simulink model "Microgrid_PV_WG_Bat_EV_j"  (R2023b)
settings: Solver=VariableStepAuto  StartTime=0.0  StopTime=1  RelTol=1e-3
undefined symbols (not defined in the file or in its folder): Acid, Ion, Lead, Lithium
libraries: slpidlib x35, spsabctodq0Lib x23, spsSeriesRLCBranchLib x19, spsCurrentMeasurementLib x13, spsVoltageMeasurementLib x11, spsThreePhaseVIMeasurementLib x10, spsPLL3phLib x9, spsThreePhaseSeriesRLCBranchLib x9, spsPower3phInstantaneousLib x8, spsIGBTDiodeLib x8, spsUniversalBridgeLib x7, spsPWMGeneratorDCDCLib x6
(part 1 of 5)
settings Model: SimulationMode=accelerator  Creator=USER  LastModifiedBy=User

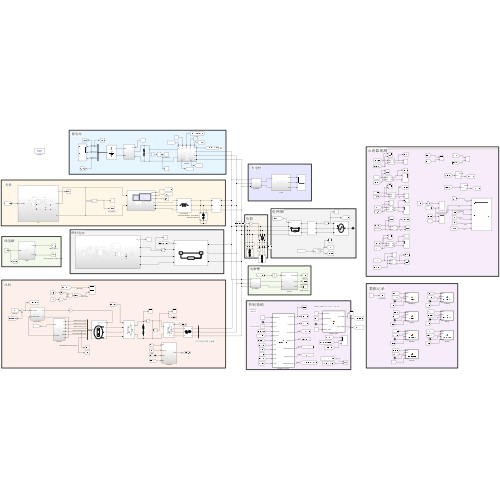
[thumbnail: Simulink's stored preview of the top-level diagram]
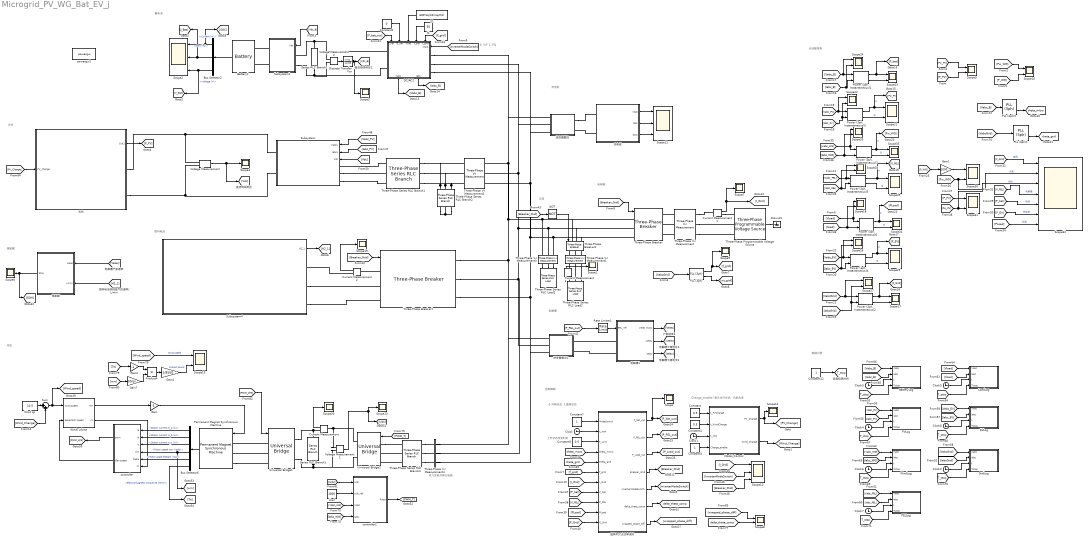
== system Microgrid_PV_WG_Bat_EV_j ==
  note: Change_enable:1表示允许光伏、风机改变
  note: :0 并网状态
      | :1 离网状态
  note: 蓄电池
  note: 储氢罐
  note: 充电桩
  note: 电解槽
  note: 燃料电池
  note: 0: V/F
      | 1: PQ
  note: 光伏
  note: 风力发电并网主电路
  note: 风机
  note: 示波器观测
  note: 数据记录
  note: 工作状态改变时刻
  note: 控制策略
  note: 负荷
  note: 电网侧
  Battery1 : spsBatteryLib/Battery  BatType=Lithium-Ion  ShowTempParam=off  ThermalPreset=no  ShowAgeParam=off  NomV=600  NomQ=10000  SOC=50  Batt_Tr=30  PresetModel=on  MaxQ=10000  MinV=450  FullV=698.3923  Dis_rate=4347.8261  R=0.0006  Normal_OP=9043.4783  expZone="[648.2315      491.3043]"  current=[6.5 13 32.5]  Units=Time  Tci=20  NomT=20  T2=-30  MaxQ2=4.8  FullV2=7.1  Normal_OP2=5.655  expZone2="[6.58           1]"  Rca=0.6  ti=2000  Dp=0  Neq0=0  Tsim=1e6  Ta1=25  Qeol=5.4*0.9  Reol=0.013333*1.2  Char_age=[2.3478, 3]  Dis_age=[2.3478, 10]  N1=1500  N2=10500  N3=1000  N4=1400  Ta2=45  N5=950
  BatteryLog : MATLAB Function  TreatAsAtomicUnit=on  SystemSampleTime=1e-5
  Bus Selector2 : BusSelector  OutputSignals=SOC (%),Current (A),Voltage (V)
  Bus Selector6 : BusSelector  OutputSignals=Stator current is_a (A),Stator current is_b (A),Stator current is_c (A),Rotor speed wm (rad/s),Rotor angle thetam (rad),Electromagnetic torque Te (N*m)
  Clock{,1..8} (9 alike) : Clock
  Constant : Constant  Value=0.5
  Constant1 : Constant  Value=0.5
  Constant12 : Constant
  Constant2 : Constant  Value=0
  Constant3 : Constant
  Constant5 : Constant  Value=0.5
  Constant7 : Constant
  Current Measurement{,1..3} (4 alike) : spsCurrentMeasurementLib/Current Measurement  PhasorSimulation=off  OutputType=Complex  PSBequivalent=0
  DC/AC2 : Subsystem
      settings: PortSchema="{\"entries\":[{\"content\":{\"sides\":[{\"content\":{\"connectorIds\":[\"LConn1\",\"LConn2\"]},\"type\":\"ConnectorPlacement.EquallySpacedRectSide\",\"uuid\":\"3c25f3ef-dfc4-4171-a66c-34d02ac02d8c\"},{\"content\":{\"connectorIds\":[\"In6\",\"RConn1\",\"RConn2\",\"RConn3\"],\"side\":\"RIGHT\"},\"type\":\"ConnectorPlacement.EquallySpacedRectSide\",\"uuid\":\"e6dce20c-09a8-4093-a340-4a6433e2abb5\"},{\"content\":{\"connectorIds\":[\"In1\",\"In2\",\"In3\",\"In4\",\"In5\"],\"side\":\"TOP\"},\"type\":\"ConnectorPlacement.EquallySpacedRectSide\",\"uuid\":\"9a728458-db9e-49f2-aa6e-65bbdb48c66f\"},{\"content\":{\"connectorIds\":[\"Out1\",\"Out2\"],\"side\":\"BOTTOM\"},\"type\":\"ConnectorPlacement.EquallySpacedRectSide\",\"uuid\":\"1b603170-02ae-4700-b32b-0d723ac1cdee\"}]},\"type\":\"ConnectorPlacement.EquallySpacedConnector\",\"uuid\":\"ee4962e9-610e-4348-91fe-b672627aeb34\"}],\"packageUris\":[\"http://schema.mathworks.com/mf0/Connector/R2020b\"],\"version\":\"1.0\"}"
  Discrete Transfer Fcn : DiscreteTransferFcn  Numerator=[0.02]  Denominator=[1 -0.98]
  EVLog : MATLAB Function  TreatAsAtomicUnit=on  SystemSampleTime=1e-5
  Gain : Gain  Gain=-1
  Gain1 : Gain  Gain=1000
  Gain2 : Gain  Gain=-1
  Gain4 : Gain  Gain=1/9550
  Gain7 : Gain  Gain=30/pi
  GridLog : MATLAB Function  TreatAsAtomicUnit=on  SystemSampleTime=1e-5
  Ground1 : spsGroundLib/Ground  LConnTagsString=a
  LoadLog : MATLAB Function  TreatAsAtomicUnit=on  SystemSampleTime=1e-5
  Model_Control : MATLAB Function  TreatAsAtomicUnit=on
  NOT : Logic  Operator=NOT  IconShape=distinctive  AllPortsSameDT=off  OutDataTypeStr=boolean
  PELLog : MATLAB Function  TreatAsAtomicUnit=on  SystemSampleTime=1e-5
  PLL (3ph) : spsPLL3phLib/PLL (3ph)  Fmin=0.0001  Par_Init=[0, 50]  ParK=[180, 3200, 1]  TcD=1e-6  MaxRateChangeFreq=100  FilterCutOffFreq=25  Ts=0  AGC=on
  PLL (3ph)1 : spsPLL3phLib/PLL (3ph)  Fmin=45  Par_Init=[0, 50]  ParK=[180, 3200, 1]  TcD=1e-4  MaxRateChangeFreq=12  FilterCutOffFreq=25  Ts=0  AGC=on
  PLL (3ph)2 : spsPLL3phLib/PLL (3ph)  Fmin=45  Par_Init=[0, 50]  ParK=[180, 3200, 1]  TcD=1e-4  MaxRateChangeFreq=12  FilterCutOffFreq=25  Ts=0  AGC=on
  PVLog : MATLAB Function  TreatAsAtomicUnit=on  SystemSampleTime=1e-5
  Permanent Magnet Synchronous Machine : spsPermanentMagnetSynchronousMachineLib/Permanent Magnet Synchronous Machine  NbPhases=3  FluxDistribution=Sinusoidal  RotorType=Round  MechanicalLoad=Torque Tm  PresetModel=No  ShowDetailedParameters=on  MeasurementBus=off  Resistance=0.025  Inductance=8.5e-3  dqInductances=[8.5e-3,8.5e-3]  La=0.0036  MachineConstant=Flux linkage established by magnets (V.s)  Flux=3.88889  VoltageCst=8464.3995  TorqueCst=70  Flat=120  Mechanical=[60 0.078 12]  PolePairs=4  InitialConditions=[0,0, 0,0]  InitialConditions5ph=[0 0 0 0 0 0]  RefAngle=90 degrees behind phase A axis (modified Park)  IterativeDiscreteModel=Trapezoidal non iterative  TsBlock=-1  TsPowergui=0
  Power (3ph, Instantaneous){1..7} (7 alike) : spsPower3phInstantaneousLib/Power (3ph, Instantaneous)
  Product4 : Product
  Rate Limiter1 : RateLimiter  RisingSlewLimit=100e5  FallingSlewLimit=-100e5
  Scope{,1,3..7,12..13,15,20} (11 alike) : Scope
  Scope10 : Scope  NumInputPorts=3
  Scope11 : Scope  NumInputPorts=3
  Scope{8..9,16..19,21..31,33..35} (20 alike) : Scope  NumInputPorts=2
  Scope2 : Scope  NumInputPorts=3
  Scope32 : Scope  NumInputPorts=7
  Series RLC Branch1 : spsSeriesRLCBranchLib/Series RLC Branch  LConnTagsString=__new0  RConnTagsString=__new0  BranchType=RC  Resistance=0.05  Inductance=1e-3  SetiL0=off  InitialCurrent=0  Capacitance=1e-2  Setx0=on  InitialVoltage=1800  Measurements=None
  Series RLC Branch2 : spsSeriesRLCBranchLib/Series RLC Branch  LConnTagsString=__new0  RConnTagsString=__new0  BranchType=RC  Resistance=0.05  Inductance=1e-3  SetiL0=off  InitialCurrent=0  Capacitance=7e-2  Setx0=on  InitialVoltage=1000  Measurements=None
  Subsystem : Subsystem
  Subsystem1 : Subsystem
  Subsystem4 : Subsystem
  Sum : Sum  Inputs=|++
  Three-Phase Programmable Voltage Source : spsThreePhaseProgrammableVoltageSourceLib/Three-Phase Programmable Voltage Source  PositiveSequence="[600  0 50]"  VariationEntity=None  VariationType=Table of time-amplitude pairs  VariationTypeAlt=Ramp  VariationStep=-5  VariationRate=100  VariationMagnitude=0.3  VariationFrequency=2  VariationTiming=[0.5 1]  VariationPhaseA=off  Amplitudes=[1 0.8 1.2 1.0]  TimeValues=[0 0.1 0.15 0.2]  HarmonicGeneration=off  HarmonicA=[3 0.2 -25 0]  HarmonicB=[2 0.15 35 2]  Timing="[0.05  3]"  BusType=swing  Pref=0  Qref=0  Qmin=-inf  Qmax=inf
  Three-Phase Series RLC Branch1 : spsThreePhaseSeriesRLCBranchLib/Three-Phase Series RLC Branch  LConnTagsString=A|B|C  RConnTagsString=A|B|C  BranchType=L  Resistance=0.1  Inductance=3e-3  Capacitance=1e-6  Measurements=None
  Three-Phase Series RLC Branch2 : spsThreePhaseSeriesRLCBranchLib/Three-Phase Series RLC Branch  LConnTagsString=A|B|C  RConnTagsString=A|B|C  BranchType=RC  Resistance=0.01  Inductance=1e-5  Capacitance=1e-5  Measurements=None
  Three-Phase Series RLC Branch3 : spsThreePhaseSeriesRLCBranchLib/Three-Phase Series RLC Branch  LConnTagsString=A|B|C  RConnTagsString=A|B|C  BranchType=RL  Resistance=0.05  Inductance=7e-3  Capacitance=1e-6  Measurements=None
  Three-Phase Series RLC Load1 : spsThreePhaseSeriesRLCLoadLib/Three-Phase Series RLC Load  LConnTagsString=A|B|C  Configuration=Y (grounded)  NominalVoltage=380  Vabc=[600 600 600]  Vabcp=[1e3 1e3 1e3]  NominalFrequency=50  UnbalancedPower=on  ActivePower=150e3  InductivePower=0  CapacitivePower=0  Pabc=[33e4 33e4 33e4]  QLabc=[100 90 110]  QCabc=[100 90 110]  Pabcp=[10e3 9e3 11e3]  QLabcp=[100 90 110]  QCabcp=[100 90 110]  Measurements=None  LoadType=constant PQ
  Three-Phase Series RLC Load2 : spsThreePhaseSeriesRLCLoadLib/Three-Phase Series RLC Load  LConnTagsString=A|B|C  Configuration=Y (grounded)  NominalVoltage=380  Vabc=[600 600 600]  Vabcp=[1e3 1e3 1e3]  NominalFrequency=50  UnbalancedPower=on  ActivePower=150e3  InductivePower=0  CapacitivePower=0  Pabc=[41e4 41e4 41e4]  QLabc=[100 90 110]  QCabc=[100 90 110]  Pabcp=[10e3 9e3 11e3]  QLabcp=[100 90 110]  QCabcp=[100 90 110]  Measurements=None  LoadType=constant PQ
  Three-Phase V-I Measurement : spsThreePhaseVIMeasurementLib/Three-Phase V-I Measurement  VoltageMeasurement=phase-to-ground  SetLabelV=on  LabelV=VabcGrid  Vpu=off  VpuLL=off  CurrentMeasurement=yes  SetLabelI=on  LabelI=IabcGrid  Ipu=off  Pbase=100e6  Vbase=500e3  OutputType=Complex  PhasorSimulation=off  PSBequivalent=0
  Three-Phase V-I Measurement1 : spsThreePhaseVIMeasurementLib/Three-Phase V-I Measurement  VoltageMeasurement=phase-to-ground  SetLabelV=on  LabelV=Vload1  Vpu=off  VpuLL=off  CurrentMeasurement=yes  SetLabelI=on  LabelI=Iload1  Ipu=off  Pbase=100e6  Vbase=500e3  OutputType=Complex  PhasorSimulation=off  PSBequivalent=0
  Three-Phase V-I Measurement2 : spsThreePhaseVIMeasurementLib/Three-Phase V-I Measurement  VoltageMeasurement=phase-to-ground  SetLabelV=on  LabelV=Vabc_PV  Vpu=off  VpuLL=off  CurrentMeasurement=yes  SetLabelI=on  LabelI=Iabc_PV  Ipu=off  Pbase=100e6  Vbase=500e3  OutputType=Complex  PhasorSimulation=off  PSBequivalent=0
  Three-Phase V-I Measurement3 : spsThreePhaseVIMeasurementLib/Three-Phase V-I Measurement  VoltageMeasurement=phase-to-ground  SetLabelV=on  LabelV=Vload  Vpu=off  VpuLL=off  CurrentMeasurement=yes  SetLabelI=on  LabelI=Iload  Ipu=off  Pbase=100e6  Vbase=500e3  OutputType=Complex  PhasorSimulation=off  PSBequivalent=0
  Three-Phase V-I Measurement4 : spsThreePhaseVIMeasurementLib/Three-Phase V-I Measurement  VoltageMeasurement=phase-to-ground  SetLabelV=on  LabelV=Vabc_WG  Vpu=off  VpuLL=off  CurrentMeasurement=yes  SetLabelI=on  LabelI=Iabc_WG  Ipu=off  Pbase=100e6  Vbase=500e3  OutputType=Complex  PhasorSimulation=off  PSBequivalent=0
  Three-Phase Breaker : spsThreePhaseBreakerLib/Three-Phase Breaker  InitialState=closed  SwitchA=on  SwitchB=on  SwitchC=on  SwitchTimes=0.2  External=on  BreakerResistance=0.0001  SnubberResistance=1e9  SnubberCapacitance=inf  Measurements=Breaker voltages and currents
  Three-Phase Breaker1 : spsThreePhaseBreakerLib/Three-Phase Breaker  InitialState=closed  SwitchA=on  SwitchB=on  SwitchC=on  SwitchTimes=0.5  External=on  BreakerResistance=0.01  SnubberResistance=1e6  SnubberCapacitance=inf  Measurements=None
  Three-Phase Breaker2 : spsThreePhaseBreakerLib/Three-Phase Breaker  InitialState=closed  SwitchA=on  SwitchB=on  SwitchC=on  SwitchTimes=0.2  External=on  BreakerResistance=0.0001  SnubberResistance=1e9  SnubberCapacitance=inf  Measurements=Breaker voltages and currents
  Universal Bridge1 : spsUniversalBridgeLib/Universal Bridge  Arms=3  SnubberResistance=1e5  SnubberCapacitance=inf  Device=IGBT / Diodes  Ron=1e-3  Lon=0  ForwardVoltages="[  0  0  ]"  ForwardVoltage=0  GTOparameters=[ 10e-6 , 20e-6 ]  IGBTparameters=[ 1e-6 , 2e-6 ]  Measurements=None  Measurements_2=None  converterType=Rectifier
  Universal Bridge2 : spsUniversalBridgeLib/Universal Bridge  Arms=3  SnubberResistance=1e5  SnubberCapacitance=inf  Device=IGBT / Diodes  Ron=1e-3  Lon=0  ForwardVoltages="[  0  0  ]"  ForwardVoltage=0  GTOparameters=[ 10e-6 , 20e-6 ]  IGBTparameters=[ 1e-6 , 2e-6 ]  Measurements=None  Measurements_2=None  converterType=Rectifier
  Uref : Constant  Value=1800
  V1 : Constant  Value=600*sqrt(2)/sqrt(3)
  Voltage Measurement : spsVoltageMeasurementLib/Voltage Measurement  PhasorSimulation=off  OutputType=Complex  PSBequivalent=0
  Voltage Measurement1 : spsVoltageMeasurementLib/Voltage Measurement  PhasorSimulation=off  OutputType=Complex  PSBequivalent=0
  Voltage Measurement2 : spsVoltageMeasurementLib/Voltage Measurement  PhasorSimulation=off  OutputType=Complex  PSBequivalent=0
  Wind sp : Constant  Value=10.5
  WindLog : MATLAB Function  TreatAsAtomicUnit=on  SystemSampleTime=1e-5
  WindTurbine : Subsystem
  controller : Subsystem
  controller2 : Subsystem
  f1 : Constant  Value=50
  powergui1 : sps_lib/powergui  Priority=1  SimulationMode=Discrete  SampleTime=1e-6  frequency=60  Iterations=50  frequencyindice=0  Pbase=100e6  ErrMax=1e-4  UnitsV=kV  UnitsW=MW  buscounter=0  FunctionMessages=off  echomessages=off  EnableUseOfTLC=off  CurrentSourceSwitches=off  DisableSnubberDevices=off  DisableRonSwitches=off  DisableVfSwitches=off  DisplayEquations=off  AutomaticDiscreteSolvers=off  SolverType=Tustin/Backward Euler (TBE)  Interpol=off  ExternalGateDelay=off  methode=off  Ts=100  x0status=blocks  SPID=on  SwTol=0  HookPort=off  NonlinearTolerance=1e-4  nMaxIteration=100  ContinueOnMaxIteration=off  RestoreLinks=warning  ResistiveCurrentMeasurement=off  Frange=[0:2:500]  Ylog=off  Xlog=on  ShowGrid=off  save=off  variable=ZData  structure=0  ZoomFFT=off  StartTime=0.0  cycles=1  DisplayStyle=1  fundamental=60  FreqAxis=off  MaxFrequency=1000  frequencyindicesteady=1  RmsSteady=1  display=off
  储氢罐 : Subsystem
  充电桩 : Subsystem
      settings: PortSchema="{\"entries\":[{\"content\":{\"sides\":[{\"content\":{\"connectorIds\":[\"Out1\",\"Out2\",\"Out3\"]},\"type\":\"ConnectorPlacement.EquallySpacedRectSide\",\"uuid\":\"de89acf6-4bf1-40b6-9ccd-ec8106de39fd\"},{\"content\":{\"connectorIds\":[\"RConn1\",\"RConn2\"],\"side\":\"RIGHT\"},\"type\":\"ConnectorPlacement.EquallySpacedRectSide\",\"uuid\":\"d03cc6c4-9473-47ce-91a0-26eb3774d9eb\"},{\"content\":{\"side\":\"TOP\"},\"type\":\"ConnectorPlacement.EquallySpacedRectSide\",\"uuid\":\"dff31fb8-dbf6-4b34-953b-d6d002de7265\"}]},\"type\":\"ConnectorPlacement.EquallySpacedConnector\",\"uuid\":\"fa66b497-f06b-485d-a451-c3139dd511e8\"}],\"packageUris\":[\"http://schema.mathworks.com/mf0/Connector/R2020b\"],\"version\":\"1.0\"}"
  光伏 : Subsystem
  电解槽1 : Subsystem
  脱网PCC点功率调节 : MATLAB Function  TreatAsAtomicUnit=on  SystemSampleTime=1e-5
  逆变器整流 : Subsystem
      settings: RTWSystemCode=Inline
  逆变器整流1 : Subsystem
      settings: RTWSystemCode=Inline
  tag scope: T_stop=global, delta_theta_comp=global, theta_grid=global, theta_micro=global
  wires:
  Discrete Transfer Fcn/1 -> Scope3/1, [Vdc_B]
  Bus Selector2/2 -> Scope2/2, [I_Bat]  "<Current (A)>"
  [Vdc_B] -> Subsystem1/1(Vdc)
  Bus Selector2/1 -> Scope2/1, [SOC]  "<SOC (%)>"
  Voltage Measurement2/1 -> Discrete Transfer Fcn/1
  Bus Selector2/3 -> Scope2/3, [V_Bat]  "<Voltage (V)>"
  Battery1/1 -> Bus Selector2/1
  [Velec] -> 储氢罐/1(Velec)
  [H2_1] -> 储氢罐/2(L/min)
  储氢罐/1(SOH) -> Scope6/1, [SOH]
  充电桩/2(Ibat) -> Scope11/2
  充电桩/3(SOC) -> Scope11/3
  充电桩/1(Vbat) -> Scope11/1
  电解槽1/3(Ielec) -> [Ielec]
  电解槽1/1(Velec mol/s) -> [Velec]
  电解槽1/2(Uelec) -> [Uelec]
  [P_PEL_out] -> Rate Limiter1/1
  Rate Limiter1/1 -> 电解槽1/1(PEL_ref)
  Subsystem4/1(H2_1) -> [H2_1]
  [VabcGrid] -> PLL (3ph)/1
  PLL (3ph)/1 -> Scope5/1, [f_grid]
  PLL (3ph)/2 -> [wt_grid]
  Current Measurement1/1 -> Scope7/1, [I_Grid]
  [Breaker_Grid] -> Three-Phase Breaker/1
  DC/AC2/1(Vabc) -> [Vabc_B]
  f1/1 -> DC/AC2/4(f_set)
  [P_bat_out] -> DC/AC2/1(P_ref)
  [InverterModeSwitch] -> DC/AC2/6(Input)
  V1/1 -> DC/AC2/3(Vset)
  [f_grid] -> DC/AC2/5(f_grid)
  Constant2/1 -> DC/AC2/2(Q_ref)
  DC/AC2/2(Iabc) -> [Iabc_B]
  [Breaker_Grid] -> Three-Phase Breaker1/1
  Constant/1 -> Model_Control/1(t_PVChange)
  Model_Control/1(PV_Change) -> [PV_Change], Scope12/1
  Model_Control/2(Wind_Change) -> [Wind_Change]
  Current Measurement2/1 -> Scope15/1
  "Power (3ph, Instantaneous)3"/1 -> [Pw_PV], Scope21/1  "P"
  [Iabc_PV] -> Scope22/2, "Power (3ph, Instantaneous)3"/2
  "Power (3ph, Instantaneous)3"/2 -> Scope21/2  "Q"
  [Vabc_PV] -> Scope22/1, "Power (3ph, Instantaneous)3"/1
  [Iabc_B] -> Scope24/2, "Power (3ph, Instantaneous)1"/2
  [Vabc_B] -> Scope24/1, "Power (3ph, Instantaneous)1"/1
  "Power (3ph, Instantaneous)1"/2 -> Scope23/2
  "Power (3ph, Instantaneous)1"/1 -> [P_bat], Scope23/1
  [Vabc_EV] -> Scope26/1, "Power (3ph, Instantaneous)4"/1
  "Power (3ph, Instantaneous)4"/2 -> Scope25/2  "Q"
  "Power (3ph, Instantaneous)4"/1 -> [P_EV], Scope25/1  "P"
  [Iabc_EV] -> Scope26/2, "Power (3ph, Instantaneous)4"/2
  [IabcGrid] -> Scope27/2, "Power (3ph, Instantaneous)2"/2
  "Power (3ph, Instantaneous)2"/1 -> [P_Grid], Scope17/1
  [VabcGrid] -> Scope27/1, "Power (3ph, Instantaneous)2"/1
  "Power (3ph, Instantaneous)2"/2 -> Scope17/2
  "Power (3ph, Instantaneous)5"/2 -> Scope29/2  "Q"
  [Vabc_PEL] -> Scope28/1, "Power (3ph, Instantaneous)5"/1
  [Iabc_PEL] -> Scope28/2, "Power (3ph, Instantaneous)5"/2
  "Power (3ph, Instantaneous)5"/1 -> [P_PEL], Scope29/1  "P"
  [P_Grid] -> Scope32/1  "电网"
  [Pw_WG] -> Scope32/2, Scope30/2  "风机"
  [P_PEL] -> Scope32/4  "电解槽"
  [P_EV] -> Scope32/6  "充电桩"
  Gain1/1 -> Scope30/1
  [Pw_PV] -> Scope32/3, Scope31/2  "光伏"
  [P_bat] -> Scope32/5  "电池"
  [P_PV] -> Scope31/1
  [P_WG] -> Gain1/1
  "Power (3ph, Instantaneous)7"/1 -> Scope35/1, [Pw_WG]  "P"
  [Iabc_WG] -> Scope33/2, "Power (3ph, Instantaneous)7"/2
  [Vabc_WG] -> Scope33/1, "Power (3ph, Instantaneous)7"/1
  "Power (3ph, Instantaneous)7"/2 -> Scope35/2  "Q"
  [Pw_PV] -> Scope9/1
  [P_PV] -> Scope9/2
  [Pw_WG] -> Scope16/1
  [P_WG] -> Scope16/2
  "Power (3ph, Instantaneous)6"/1 -> Scope34/1, [PLoad]  "P"
  [Vload] -> Scope18/1, "Power (3ph, Instantaneous)6"/1
  [Iload] -> Scope18/2, "Power (3ph, Instantaneous)6"/2
  "Power (3ph, Instantaneous)6"/2 -> Scope34/2  "Q"
  [PLoad] -> Scope32/7  "负载"
  [PLoad] -> 脱网PCC点功率调节/10(PLoad)
  [P_Grid] -> 脱网PCC点功率调节/11(P_Grid)
  [P_bat] -> 脱网PCC点功率调节/8(P_bat)
  [P_PEL] -> 脱网PCC点功率调节/9(P_PEL)
  [I_Grid] -> Scope10/1
  [InverterModeSwitch] -> Scope10/2
  [Breaker_Grid] -> Scope10/3
  脱网PCC点功率调节/3(P_Load_out) -> [P_Load_out]
  [Iabc_PV] -> Subsystem/2(IabcL)
  [Vabc_PV] -> Subsystem/1(VabcL)
  光伏/1(Out1) -> [P_PV]
  Voltage Measurement/1 -> Scope4/1, [Vdc]
  [Vdc] -> Subsystem/3(Vdc)
  controller/2(Gen speed) -> WindTurbine/2(Generator speed)
  [Wind_Change] -> Sum/2
  Current Measurement/1 -> Scope20/1
  Bus Selector6/6 -> [Te]  "<Electromagnetic torque Te (N*m)>"
  [Iabc_WG] -> controller2/4(Iabc)
  Voltage Measurement1/1 -> [Udc], Scope13/1
  Gain/1 -> Permanent Magnet Synchronous Machine/1
  [Udc] -> controller2/1(Udc)
  Bus Selector6/3 -> controller/3(ic)  "<Stator current is_c (A)>"
  Gain4/1 -> Scope19/2  "Output power"
  WindTurbine/1(Tm) -> Gain/1
  [Vabc_WG] -> controller2/3(Vabc)
  Bus Selector6/4 -> [wm], controller/4(wm)  "<Rotor speed wm (rad/s)>"
  Permanent Magnet Synchronous Machine/1 -> Bus Selector6/1
  Gain7/1 -> Product4/2
  [PWM_T] -> Universal Bridge2/1
  Sum/1 -> WindTurbine/1(Wind speed), [Wind_speed]
  controller/1(pwm) -> [PWM_WG]
  [PWM_WG] -> Universal Bridge1/1
  [wm] -> Gain7/1
  [Wind_speed] -> Scope19/1  "Wind speed"
  Bus Selector6/1 -> controller/1(ia)  "<Stator current is_a (A)>"
  Gain2/1 -> Product4/1
  Bus Selector6/5 -> controller/5(theta)  "<Rotor angle thetam (rad)>"
  Bus Selector6/2 -> controller/2(ib)  "<Stator current is_b (A)>"
  WindTurbine/2(n*) -> controller/6(n*)
  Wind sp/1 -> Sum/1
  Product4/1 -> Gain4/1
  controller2/1(Pulse) -> [PWM_T]
  [Te] -> Gain2/1
  Uref/1 -> controller2/2(Udc_ref)
  [I_Grid] -> 脱网PCC点功率调节/7(I_Grid)
  [f_grid] -> 脱网PCC点功率调节/6(f_grid)
  脱网PCC点功率调节/4(Breaker_Grid) -> [Breaker_Grid]
  脱网PCC点功率调节/5(InverterModeSwitch) -> [InverterModeSwitch]
  Constant7/1 -> 脱网PCC点功率调节/1(ModeSwitch)
  脱网PCC点功率调节/6(delta_theta_comp) -> [delta_theta_comp]
  Constant5/1 -> 脱网PCC点功率调节/3(t_sync)
  [theta_micro] -> 脱网PCC点功率调节/4(theta_micro)
  [theta_grid] -> 脱网PCC点功率调节/5(theta_grid)
  Clock/1 -> 脱网PCC点功率调节/2(t_now)
  脱网PCC点功率调节/2(P_PEL_out) -> [P_PEL_out]
  脱网PCC点功率调节/1(P_bat_out) -> Scope/1, [P_bat_out]
  [VabcGrid] -> GridLog/1(Vabc)
  [IabcGrid] -> GridLog/2(Iabc)
  Clock2/1 -> GridLog/3(t)
  [T_stop] -> GridLog/4(Tstop)
  [T_stop] -> BatteryLog/4(Tstop)
  [Vabc_B] -> BatteryLog/1(Vabc)
  [Iabc_B] -> BatteryLog/2(Iabc)
  Clock3/1 -> BatteryLog/3(t)
  [T_stop] -> PVLog/4(Tstop)
  [Vabc_PV] -> PVLog/1(Vabc)
  [Iabc_PV] -> PVLog/2(Iabc)
  Clock4/1 -> PVLog/3(t)
  [T_stop] -> LoadLog/4(Tstop)
  [Vload] -> LoadLog/1(Vabc)
  [Iload] -> LoadLog/2(Iabc)
  Clock5/1 -> LoadLog/3(t)
  [T_stop] -> WindLog/4(Tstop)
  [Vabc_WG] -> WindLog/1(Vabc)
  [Iabc_WG] -> WindLog/2(Iabc)
  Clock6/1 -> WindLog/3(t)
  [T_stop] -> PELLog/4(Tstop)
  [Vabc_PEL] -> PELLog/1(Vabc)
  [Iabc_PEL] -> PELLog/2(Iabc)
  Clock7/1 -> PELLog/3(t)
  [T_stop] -> EVLog/4(Tstop)
  [Vabc_EV] -> EVLog/1(Vabc)
  [Iabc_EV] -> EVLog/2(Iabc)
  Clock8/1 -> EVLog/3(t)
  Constant12/1 -> [T_stop]
  NOT/1 -> Three-Phase Breaker2/1
  Current Measurement3/1 -> Scope1/1
  [Breaker_Grid] -> NOT/1
  [Vabc_B] -> PLL (3ph)2/1
  PLL (3ph)2/2 -> [theta_micro]
  PLL (3ph)1/2 -> [theta_grid]
  [VabcGrid] -> PLL (3ph)1/1
  脱网PCC点功率调节/7(wrapped_phase_diff) -> [wrapped_phase_diff]
  [delta_theta_comp] -> Scope8/2
  [wrapped_phase_diff] -> Scope8/1
  Clock1/1 -> Model_Control/3(t_now)
  Constant1/1 -> Model_Control/2(t_WindChange)
  [PV_Change] -> 光伏/1(PV_change)
  Constant3/1 -> Model_Control/4(Change_enable)
  connections:
  Three-Phase V-I Measurement/LConn3 -- Three-Phase Programmable Voltage Source/RConn3
  Three-Phase V-I Measurement/LConn2 -- Three-Phase Programmable Voltage Source/RConn2
  Three-Phase V-I Measurement3/LConn2 -- Three-Phase Series RLC Load1/LConn2
  Three-Phase V-I Measurement3/LConn1 -- Three-Phase Series RLC Load1/LConn1
  Three-Phase V-I Measurement3/LConn3 -- Three-Phase Series RLC Load1/LConn3
  Series RLC Branch2/LConn1 -- DC/AC2/LConn1 -- Voltage Measurement2/LConn1 -- Subsystem1/LConn1
  Subsystem1/LConn2 -- Series RLC Branch2/RConn1 -- DC/AC2/LConn2 -- Voltage Measurement2/LConn2
  Subsystem1/RConn1 -- Battery1/LConn1
  Subsystem1/RConn2 -- Battery1/LConn2
  逆变器整流/LConn1 -- 充电桩/RConn1
  充电桩/RConn2 -- 逆变器整流/LConn2
  电解槽1/LConn1 -- 逆变器整流1/LConn1
  电解槽1/LConn2 -- 逆变器整流1/LConn2
  Subsystem4/RConn2 -- Three-Phase Breaker1/LConn2
  Subsystem4/RConn3 -- Three-Phase Breaker1/LConn3
  Three-Phase V-I Measurement/RConn1 -- Three-Phase Breaker/RConn1
  Three-Phase V-I Measurement/RConn2 -- Three-Phase Breaker/RConn2
  Three-Phase V-I Measurement/RConn3 -- Three-Phase Breaker/RConn3
  Three-Phase Programmable Voltage Source/LConn1 -- Ground1/LConn1
  Three-Phase V-I Measurement/LConn1 -- Current Measurement1/LConn1
  Current Measurement1/RConn1 -- Three-Phase Programmable Voltage Source/RConn1
  Three-Phase Breaker1/LConn1 -- Current Measurement2/LConn1
  Current Measurement2/RConn1 -- Subsystem4/RConn1
  Voltage Measurement/LConn2 -- 光伏/RConn2 -- Subsystem/RConn2
  Voltage Measurement/LConn1 -- 光伏/RConn1 -- Subsystem/RConn1
  Three-Phase Series RLC Branch2/LConn3 -- Three-Phase V-I Measurement2/LConn3 -- Three-Phase Series RLC Branch1/RConn3
  Three-Phase Series RLC Branch2/LConn1 -- Three-Phase V-I Measurement2/LConn1 -- Three-Phase Series RLC Branch1/RConn1
  Three-Phase Series RLC Branch2/LConn2 -- Three-Phase V-I Measurement2/LConn2 -- Three-Phase Series RLC Branch1/RConn2
  Subsystem/LConn2 -- Three-Phase Series RLC Branch1/LConn2
  Three-Phase Series RLC Branch1/LConn1 -- Subsystem/LConn1
  Subsystem/LConn3 -- Three-Phase Series RLC Branch1/LConn3
  DC/AC2/RConn1 -- 逆变器整流/RConn1 -- Three-Phase V-I Measurement2/RConn1 -- Three-Phase V-I Measurement4/RConn1 -- 逆变器整流1/RConn1 -- Three-Phase Breaker1/RConn1 -- Three-Phase Breaker2/LConn1 -- Three-Phase Breaker/LConn1 -- Three-Phase V-I Measurement3/RConn1
  DC/AC2/RConn2 -- 逆变器整流/RConn2 -- Three-Phase V-I Measurement4/RConn2 -- 逆变器整流1/RConn2 -- Three-Phase Breaker1/RConn2 -- Three-Phase Breaker2/LConn2 -- Three-Phase Breaker/LConn2 -- Three-Phase V-I Measurement3/RConn2 -- Three-Phase V-I Measurement2/RConn2
  Three-Phase Breaker1/RConn3 -- Three-Phase V-I Measurement4/RConn3 -- 逆变器整流1/RConn3 -- DC/AC2/RConn3 -- 逆变器整流/RConn3 -- Three-Phase V-I Measurement2/RConn3 -- Three-Phase Breaker2/LConn3 -- Three-Phase Breaker/LConn3 -- Three-Phase V-I Measurement3/RConn3
  Three-Phase Series RLC Branch2/RConn1 -- Three-Phase Series RLC Branch2/RConn3 -- Three-Phase Series RLC Branch2/RConn2
  Current Measurement/LConn1 -- Voltage Measurement1/LConn1 -- Universal Bridge2/RConn1
  Series RLC Branch1/RConn1 -- Universal Bridge2/RConn2 -- Voltage Measurement1/LConn2 -- Universal Bridge1/RConn2
  Universal Bridge1/RConn1 -- Series RLC Branch1/LConn1 -- Current Measurement/RConn1
  Three-Phase Series RLC Branch3/LConn3 -- Universal Bridge2/LConn3
  Three-Phase Series RLC Branch3/RConn2 -- Three-Phase V-I Measurement4/LConn2
  Universal Bridge1/LConn2 -- Permanent Magnet Synchronous Machine/LConn2
  Universal Bridge1/LConn1 -- Permanent Magnet Synchronous Machine/LConn1
  Universal Bridge2/LConn1 -- Three-Phase Series RLC Branch3/LConn1
  Three-Phase Series RLC Branch3/RConn1 -- Three-Phase V-I Measurement4/LConn1
  Three-Phase Series RLC Branch3/LConn2 -- Universal Bridge2/LConn2
  Permanent Magnet Synchronous Machine/LConn3 -- Universal Bridge1/LConn3
  Three-Phase Series RLC Branch3/RConn3 -- Three-Phase V-I Measurement4/LConn3
  Three-Phase Series RLC Load2/LConn2 -- Three-Phase V-I Measurement1/LConn2
  Three-Phase Series RLC Load2/LConn3 -- Three-Phase V-I Measurement1/LConn3
  Three-Phase V-I Measurement1/RConn1 -- Three-Phase Breaker2/RConn1
  Three-Phase V-I Measurement1/RConn2 -- Three-Phase Breaker2/RConn2
  Three-Phase V-I Measurement1/RConn3 -- Three-Phase Breaker2/RConn3
  Current Measurement3/RConn1 -- Three-Phase V-I Measurement1/LConn1
  Three-Phase Series RLC Load2/LConn1 -- Current Measurement3/LConn1

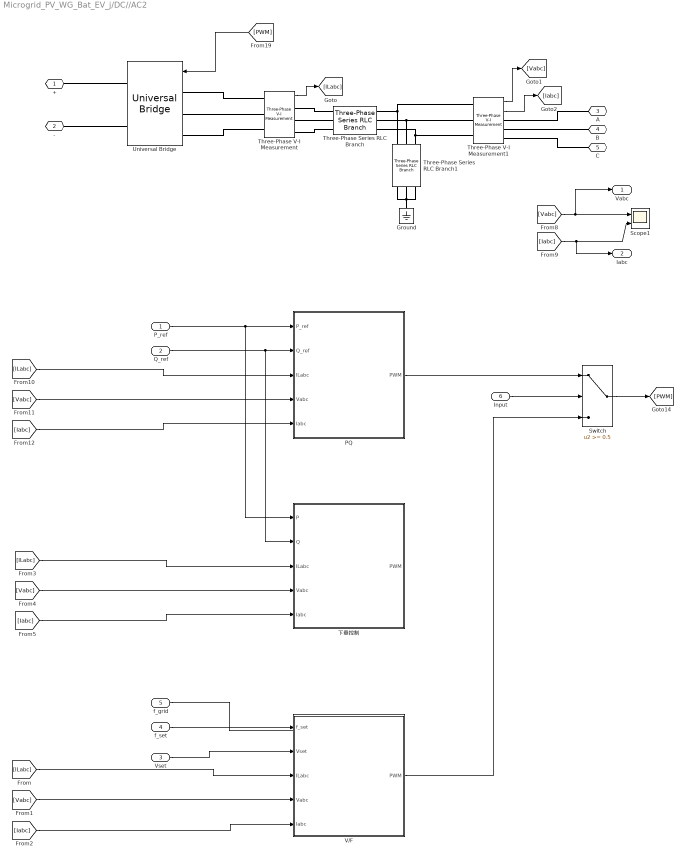
== system Microgrid_PV_WG_Bat_EV_j/DC//AC2 ==
  P_ref : Inport
  Q_ref : Inport  Port=2
  Vset : Inport  Port=3
  f_set : Inport  Port=4
  f_grid : Inport  Port=5
  Input : Inport  Port=6
  Ground : spsGroundLib/Ground  LConnTagsString=a
  PQ : Subsystem
  Scope1 : Scope  NumInputPorts=2
  Switch : Switch  Threshold=0.5  SaturateOnIntegerOverflow=off  InputSameDT=off
  Three-Phase Series RLC Branch : spsThreePhaseSeriesRLCBranchLib/Three-Phase Series RLC Branch  LConnTagsString=A|B|C  RConnTagsString=A|B|C  BranchType=RL  Resistance=1e-5  Inductance=3e-3  Capacitance=1e-6  Measurements=None
  Three-Phase Series RLC Branch1 : spsThreePhaseSeriesRLCBranchLib/Three-Phase Series RLC Branch  LConnTagsString=A|B|C  RConnTagsString=A|B|C  BranchType=RC  Resistance=0.01  Inductance=1e-3  Capacitance=20e-6  Measurements=None
  Three-Phase V-I Measurement : spsThreePhaseVIMeasurementLib/Three-Phase V-I Measurement  VoltageMeasurement=no  SetLabelV=off  LabelV=Vabc  Vpu=off  VpuLL=off  CurrentMeasurement=yes  SetLabelI=off  LabelI=ILabc  Ipu=off  Pbase=100e6  Vbase=500e3  OutputType=Complex  PhasorSimulation=off  PSBequivalent=0
  Three-Phase V-I Measurement1 : spsThreePhaseVIMeasurementLib/Three-Phase V-I Measurement  VoltageMeasurement=phase-to-ground  SetLabelV=off  LabelV=Vabc  Vpu=off  VpuLL=off  CurrentMeasurement=yes  SetLabelI=off  LabelI=Iabc  Ipu=off  Pbase=100e6  Vbase=500e3  OutputType=Complex  PhasorSimulation=off  PSBequivalent=0
  Universal Bridge : spsUniversalBridgeLib/Universal Bridge  Arms=3  SnubberResistance=1e5  SnubberCapacitance=inf  Device=IGBT / Diodes  Ron=1e-3  Lon=0  ForwardVoltages="[  0  0  ]"  ForwardVoltage=0  GTOparameters=[ 10e-6 , 20e-6 ]  IGBTparameters=[ 1e-6 , 2e-6 ]  Measurements=None  Measurements_2=None  converterType=Rectifier
  V/F : Subsystem
  下垂控制 : Subsystem
  + : PMIOPort  Side=Left
  - : PMIOPort  Port=2  Side=Left
  A : PMIOPort  Port=3  Side=Right
  B : PMIOPort  Port=4  Side=Right
  C : PMIOPort  Port=5  Side=Right
  Vabc : Outport
  Iabc : Outport  Port=2
  wires:
  Three-Phase V-I Measurement1/1 -> [Vabc]
  Three-Phase V-I Measurement/1 -> [ILabc]
  Three-Phase V-I Measurement1/2 -> [Iabc]
  [PWM] -> Universal Bridge/1
  Vset/1 -> V/F/2(Vset)
  [Vabc] -> PQ/4(Vabc)
  [Iabc] -> PQ/5(Iabc)
  [Vabc] -> V/F/4(Vabc)
  [Iabc] -> V/F/5(Iabc)
  [ILabc] -> V/F/3(ILabc)
  [ILabc] -> PQ/3(ILabc)
  [Iabc] -> Iabc/1, Scope1/2
  [Vabc] -> Vabc/1, Scope1/1
  Switch/1 -> [PWM]
  Input/1 -> Switch/2
  f_grid/1 -> ?
  f_set/1 -> V/F/1(f_set)
  [ILabc] -> 下垂控制/3(ILabc)
  [Vabc] -> 下垂控制/4(Vabc)
  Q_ref/1 -> 下垂控制/2(Q), PQ/2(Q_ref)
  P_ref/1 -> 下垂控制/1(P), PQ/1(P_ref)
  [Iabc] -> 下垂控制/5(Iabc)
  PQ/1(PWM) -> Switch/1
  V/F/1(PWM) -> Switch/3
  connections:
  Universal Bridge/LConn3 -- Three-Phase V-I Measurement/LConn3
  Three-Phase Series RLC Branch/RConn2 -- Three-Phase V-I Measurement1/LConn2 -- Three-Phase Series RLC Branch1/LConn2
  Universal Bridge/LConn1 -- Three-Phase V-I Measurement/LConn1
  Three-Phase V-I Measurement1/RConn2 -- B/RConn1
  +/RConn1 -- Universal Bridge/RConn1
  Three-Phase Series RLC Branch/RConn3 -- Three-Phase V-I Measurement1/LConn3 -- Three-Phase Series RLC Branch1/LConn3
  Three-Phase Series RLC Branch/LConn2 -- Three-Phase V-I Measurement/RConn2
  A/RConn1 -- Three-Phase V-I Measurement1/RConn1
  Ground/LConn1 -- Three-Phase Series RLC Branch1/RConn2 -- Three-Phase Series RLC Branch1/RConn3 -- Three-Phase Series RLC Branch1/RConn1
  Three-Phase Series RLC Branch1/LConn1 -- Three-Phase V-I Measurement1/LConn1 -- Three-Phase Series RLC Branch/RConn1
  -/RConn1 -- Universal Bridge/RConn2
  Three-Phase Series RLC Branch/LConn1 -- Three-Phase V-I Measurement/RConn1
  C/RConn1 -- Three-Phase V-I Measurement1/RConn3
  Universal Bridge/LConn2 -- Three-Phase V-I Measurement/LConn2
  Three-Phase Series RLC Branch/LConn3 -- Three-Phase V-I Measurement/RConn3

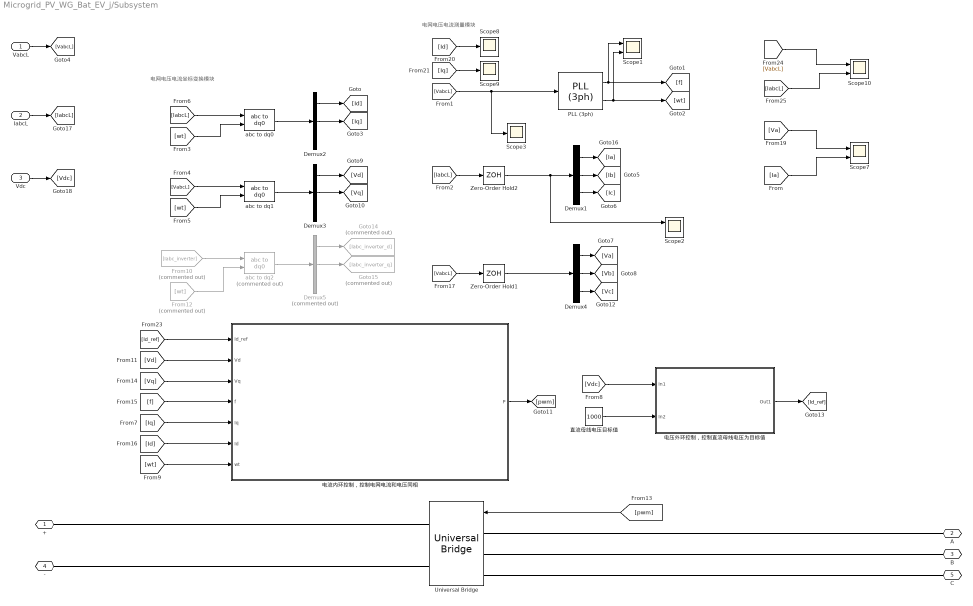
== system Microgrid_PV_WG_Bat_EV_j/Subsystem ==
  note: 电网电压电流坐标变换模块
  note: 电网电压电流测量模块
  VabcL : Inport
  IabcL : Inport  Port=2
  Vdc : Inport  Port=3
  Demux{1..4} (4 alike) : Demux  Outputs=3
  Demux5 : Demux  Commented=on  Outputs=3
  From10 : From  Commented=on  GotoTag=Iabc_inverter  TagVisibility=global
  From12 : From  Commented=on  GotoTag=wt
  Goto14 : Goto  Commented=on  GotoTag=Iabc_inverter_d
  Goto15 : Goto  Commented=on  GotoTag=Iabc_inverter_q
  PLL (3ph) : spsPLL3phLib/PLL (3ph)  Fmin=45  Par_Init=[0, 50]  ParK=[180, 3200, 1]  TcD=1e-4  MaxRateChangeFreq=12  FilterCutOffFreq=25  Ts=0  AGC=on
  Scope{1..2,7,10} (4 alike) : Scope  NumInputPorts=2
  Scope3 : Scope
  Scope8 : Scope
  Scope9 : Scope
  Universal Bridge : spsUniversalBridgeLib/Universal Bridge  Arms=3  SnubberResistance=1e5  SnubberCapacitance=inf  Device=MOSFET / Diodes  Ron=1e-3  Lon=0  ForwardVoltages="[  0  0  ]"  ForwardVoltage=0  GTOparameters=[ 10e-6 , 20e-6 ]  IGBTparameters=[ 1e-6 , 2e-6 ]  Measurements=None  Measurements_2=None  converterType=Rectifier
  Zero-Order Hold1 : ZeroOrderHold  SampleTime=-1
  Zero-Order Hold2 : ZeroOrderHold  SampleTime=-1
  abc to dq0 : spsabctodq0Lib/abc to dq0  Alignment=90 degrees behind phase A axis
  abc to dq1 : spsabctodq0Lib/abc to dq0  Alignment=90 degrees behind phase A axis
  abc to dq2 : spsabctodq0Lib/abc to dq0  Commented=on  Alignment=90 degrees behind phase A axis
  电压外环控制，控制直流母线电压为目标值 : Subsystem
  电流内环控制，控制电网电流和电压同相 : Subsystem
  直流母线电压目标值 : Constant  Value=1000
  + : PMIOPort  Side=Right
  A : PMIOPort  Port=2  Side=Left
  B : PMIOPort  Port=3  Side=Left
  - : PMIOPort  Port=4  Side=Right
  C : PMIOPort  Port=5  Side=Left
  wires:
  Demux4/2 -> [Vb]
  [Vdc] -> 电压外环控制，控制直流母线电压为目标值/1(In1)
  [Va] -> Scope7/1
  Demux3/2 -> [Vq]
  Demux1/2 -> [Ib]
  [VabcL] -> Scope10/1
  [Iq] -> Scope9/1
  Demux3/1 -> [Vd]
  [Id_ref] -> 电流内环控制，控制电网电流和电压同相/1(Id_ref)
  abc to dq2/1 -> Demux5/1
  [Id] -> Scope8/1
  [wt] -> abc to dq0/2
  Demux4/1 -> [Va]
  PLL (3ph)/1 -> [f], Scope1/1
  Zero-Order Hold2/1 -> Scope2/1, Demux1/1
  Demux1/3 -> [Ic]
  [Id] -> 电流内环控制，控制电网电流和电压同相/6(Id)
  Demux1/1 -> [Ia]
  [IabcL] -> abc to dq0/1
  [Vd] -> 电流内环控制，控制电网电流和电压同相/2(Vd)
  Demux4/3 -> [Vc]
  Demux2/1 -> [Id]
  [VabcL] -> abc to dq1/1
  直流母线电压目标值/1 -> 电压外环控制，控制直流母线电压为目标值/2(In2)
  abc to dq0/1 -> Demux2/1
  abc to dq1/1 -> Demux3/1
  Demux2/2 -> [Iq]
  [Ia] -> Scope7/2
  [wt] -> abc to dq1/2
  [wt] -> 电流内环控制，控制电网电流和电压同相/7(wt)
  [f] -> 电流内环控制，控制电网电流和电压同相/4(f)
  Demux5/2 -> Goto15/1
  [IabcL] -> Scope10/2
  电流内环控制，控制电网电流和电压同相/1(P) -> [pwm]
  [Vq] -> 电流内环控制，控制电网电流和电压同相/3(Vq)
  [pwm] -> Universal Bridge/1
  [Iq] -> 电流内环控制，控制电网电流和电压同相/5(Iq)
  电压外环控制，控制直流母线电压为目标值/1(Out1) -> [Id_ref]
  Demux5/1 -> Goto14/1
  PLL (3ph)/2 -> [wt], Scope1/2
  From10/1 -> abc to dq2/1
  From12/1 -> abc to dq2/2
  [VabcL] -> Scope3/1, PLL (3ph)/1
  [IabcL] -> Zero-Order Hold2/1
  [VabcL] -> Zero-Order Hold1/1
  Zero-Order Hold1/1 -> Demux4/1
  VabcL/1 -> [VabcL]
  IabcL/1 -> [IabcL]
  Vdc/1 -> [Vdc]
  connections:
  Universal Bridge/LConn2 -- B/RConn1
  +/RConn1 -- Universal Bridge/RConn1
  Universal Bridge/LConn3 -- C/RConn1
  Universal Bridge/RConn2 -- -/RConn1
  Universal Bridge/LConn1 -- A/RConn1

== system Microgrid_PV_WG_Bat_EV_j/Subsystem1 ==
  Vdc : Inport
  Add1 : Sum  Inputs=+-
  Add2 : Sum  Inputs=+-
  Constant2 : Constant  Value=2000
  Current Measurement1 : spsCurrentMeasurementLib/Current Measurement  PhasorSimulation=off  OutputType=Complex  PSBequivalent=0
  IGBT/Diode : spsIGBTDiodeLib/IGBT//Diode  Ron=1e-3  Rs=1e5  Cs=inf  Measurements=on
  IGBT/Diode1 : spsIGBTDiodeLib/IGBT//Diode  Ron=1e-3  Rs=1e5  Cs=inf  Measurements=on
  NOT1 : Logic  Operator=NOT  IconShape=distinctive  AllPortsSameDT=off  OutDataTypeStr=boolean
  PID Controller1 : slpidlib/PID Controller  Controller=PI  Form=Parallel  TimeDomain=Discrete-time  UseExternalTs=off  SampleTime=1e-5  IntegratorMethod=Forward Euler  FilterMethod=Forward Euler  ControllerParametersSource=internal  P=1  I=1  UseKiTs=off  D=0  N=100  UseFilter=on  TunerSelectOption=Transfer Function Based (PID Tuner App)  InitialConditionSource=internal  InitialConditionForIntegrator=0  InitialConditionForFilter=0  DifferentiatorICPrevScaledInput=0  ExternalReset=none  TrackingMode=off  Kt=1  LimitOutput=off  SatLimitsSource=internal  UpperSaturationLimit=inf  LowerSaturationLimit=-inf  LinearizeAsGain=on  AntiWindupMode=none  Kb=1  LimitIntegrator=off  UpperIntegratorSaturationLimit=inf  LowerIntegratorSaturationLimit=-inf  POutMin=[]  POutMax=[]  IOutMin=[]  IOutMax=[]  DOutMin=[]  DOutMax=[]  NOutMin=[]  NOutMax=[]  SumOutMin=[]  SumOutMax=[]  SaturationOutMin=[]  SaturationOutMax=[]  PParamMin=[]  PParamMax=[]  IParamMin=[]  IParamMax=[]  DParamMin=[]  DParamMax=[]  NParamMin=[]  NParamMax=[]  KbParamMin=[]  KbParamMax=[]  KtParamMin=[]  KtParamMax=[]  KbOutMin=[]  KbOutMax=[]  KtOutMin=[]  KtOutMax=[]  IntegratorOutMin=[]  IntegratorOutMax=[]  FilterOutMin=[]  FilterOutMax=[]  SumI1OutMin=[]  SumI1OutMax=[]  SumI2OutMin=[]  SumI2OutMax=[]  SumI3OutMin=[]  SumI3OutMax=[]  SumI4OutMin=[]  SumI4OutMax=[]  SumDOutMin=[]  SumDOutMax=[]  DifferentiatorOutMin=[]  DifferentiatorOutMax=[]  FilterDiffOutCoefMin=[]  FilterDiffOutCoefMax=[]  ReciprocalOutMin=[]  ReciprocalOutMax=[]  SumDenOutMin=[]  SumDenOutMax=[]  SumNumOutMin=[]  SumNumOutMax=[]  DivideOutMin=[]  DivideOutMax=[]  UdiffTsProdOutMin=[]  UdiffTsProdOutMax=[]  NTsProdOutMin=[]  NTsProdOutMax=[]  UintegralTsProdOutMin=[]  UintegralTsProdOutMax=[]  UngainTsProdOutMin=[]  UngainTsProdOutMax=[]  ClampingZeroOutDataTypeStr=Inherit: Inherit via back propagation  ClampingZeroOutMin=[]  ClampingZeroOutMax=[]  FilterDenConstantOutDataTypeStr=Inherit: Inherit via back propagation  FilterDenConstantOutMin=[]  FilterDenConstantOutMax=[]  PCopyOutDataTypeStr=Inherit: Inherit via back propagation  PCopyOutMin=[]  PCopyOutMax=[]  NCopyOutDataTypeStr=Inherit: Inherit via back propagation  NCopyOutMin=[]  NCopyOutMax=[]  IntegratorContinuousStateAttributes=''  IntegratorStateMustResolveToSignalObject=off  IntegratorRTWStateStorageClass=Auto  FilterContinuousStateAttributes=''  FilterStateMustResolveToSignalObject=off  FilterRTWStateStorageClass=Auto  ParallelPVariant=InternalParameters  IdealPVariant=Disabled  IVariant=InternalParameters  DVariant=Disabled  IntegratorVariant=Discrete  SatVariant=Disabled  AWVariant=Passthrough  PCopyVariant=Disabled  TRVariant=Disabled  FdbkBlocksVariant=Forward  IdealPFdbkVariant=Disabled  SatFdbkVariant=Disabled  DerivativeFilterVariant=Disabled  NVariant=Disabled  NCopyVariant=Disabled_SignalSpec  FilterICVariant=Disabled  IntegratorICVariant=InternalICs  ExternalResetVariant=Disabled  TRSumVariant=Passthrough  SumFdbkVariant=Disabled  SumVariant=Sum_PI  TsampFilterVariant=InternalTs  TsampNgainVariant=Passthrough  TsampIntegralVariant=Disabled_SignalSpec  ExternalSaturationOutDataTypeStr=Inherit: Same as second input
  PID Controller2 : slpidlib/PID Controller  Controller=PI  Form=Parallel  TimeDomain=Discrete-time  UseExternalTs=off  SampleTime=1e-5  IntegratorMethod=Forward Euler  FilterMethod=Forward Euler  ControllerParametersSource=internal  P=5  I=10  UseKiTs=off  D=0  N=100  UseFilter=on  TunerSelectOption=Transfer Function Based (PID Tuner App)  InitialConditionSource=internal  InitialConditionForIntegrator=0  InitialConditionForFilter=0  DifferentiatorICPrevScaledInput=0  ExternalReset=none  TrackingMode=off  Kt=1  LimitOutput=off  SatLimitsSource=internal  UpperSaturationLimit=inf  LowerSaturationLimit=-inf  LinearizeAsGain=on  AntiWindupMode=none  Kb=1  LimitIntegrator=off  UpperIntegratorSaturationLimit=inf  LowerIntegratorSaturationLimit=-inf  POutMin=[]  POutMax=[]  IOutMin=[]  IOutMax=[]  DOutMin=[]  DOutMax=[]  NOutMin=[]  NOutMax=[]  SumOutMin=[]  SumOutMax=[]  SaturationOutMin=[]  SaturationOutMax=[]  PParamMin=[]  PParamMax=[]  IParamMin=[]  IParamMax=[]  DParamMin=[]  DParamMax=[]  NParamMin=[]  NParamMax=[]  KbParamMin=[]  KbParamMax=[]  KtParamMin=[]  KtParamMax=[]  KbOutMin=[]  KbOutMax=[]  KtOutMin=[]  KtOutMax=[]  IntegratorOutMin=[]  IntegratorOutMax=[]  FilterOutMin=[]  FilterOutMax=[]  SumI1OutMin=[]  SumI1OutMax=[]  SumI2OutMin=[]  SumI2OutMax=[]  SumI3OutMin=[]  SumI3OutMax=[]  SumI4OutMin=[]  SumI4OutMax=[]  SumDOutMin=[]  SumDOutMax=[]  DifferentiatorOutMin=[]  DifferentiatorOutMax=[]  FilterDiffOutCoefMin=[]  FilterDiffOutCoefMax=[]  ReciprocalOutMin=[]  ReciprocalOutMax=[]  SumDenOutMin=[]  SumDenOutMax=[]  SumNumOutMin=[]  SumNumOutMax=[]  DivideOutMin=[]  DivideOutMax=[]  UdiffTsProdOutMin=[]  UdiffTsProdOutMax=[]  NTsProdOutMin=[]  NTsProdOutMax=[]  UintegralTsProdOutMin=[]  UintegralTsProdOutMax=[]  UngainTsProdOutMin=[]  UngainTsProdOutMax=[]  ClampingZeroOutDataTypeStr=Inherit: Inherit via back propagation  ClampingZeroOutMin=[]  ClampingZeroOutMax=[]  FilterDenConstantOutDataTypeStr=Inherit: Inherit via back propagation  FilterDenConstantOutMin=[]  FilterDenConstantOutMax=[]  PCopyOutDataTypeStr=Inherit: Inherit via back propagation  PCopyOutMin=[]  PCopyOutMax=[]  NCopyOutDataTypeStr=Inherit: Inherit via back propagation  NCopyOutMin=[]  NCopyOutMax=[]  IntegratorContinuousStateAttributes=''  IntegratorStateMustResolveToSignalObject=off  IntegratorRTWStateStorageClass=Auto  FilterContinuousStateAttributes=''  FilterStateMustResolveToSignalObject=off  FilterRTWStateStorageClass=Auto  ParallelPVariant=InternalParameters  IdealPVariant=Disabled  IVariant=InternalParameters  DVariant=Disabled  IntegratorVariant=Discrete  SatVariant=Disabled  AWVariant=Passthrough  PCopyVariant=Disabled  TRVariant=Disabled  FdbkBlocksVariant=Forward  IdealPFdbkVariant=Disabled  SatFdbkVariant=Disabled  DerivativeFilterVariant=Disabled  NVariant=Disabled  NCopyVariant=Disabled_SignalSpec  FilterICVariant=Disabled  IntegratorICVariant=InternalICs  ExternalResetVariant=Disabled  TRSumVariant=Passthrough  SumFdbkVariant=Disabled  SumVariant=Sum_PI  TsampFilterVariant=InternalTs  TsampNgainVariant=Passthrough  TsampIntegralVariant=Disabled_SignalSpec  ExternalSaturationOutDataTypeStr=Inherit: Same as second input
  PWM Generator (DC-DC)2 : spsPWMGeneratorDCDCLib/PWM Generator (DC-DC)  Fsw=1e4  Ts=0
  Scope1 : Scope
  Scope13 : Scope
  Series RLC Branch2 : spsSeriesRLCBranchLib/Series RLC Branch  LConnTagsString=__new0  RConnTagsString=__new0  BranchType=L  Resistance=1  Inductance=8e-3  SetiL0=off  InitialCurrent=0  Capacitance=1e-6  Setx0=off  InitialVoltage=0  Measurements=None
  Series RLC Branch4 : spsSeriesRLCBranchLib/Series RLC Branch  LConnTagsString=__new0  RConnTagsString=__new0  BranchType=C  Resistance=1  Inductance=1e-3  SetiL0=off  InitialCurrent=0  Capacitance=1e-2  Setx0=on  InitialVoltage=600  Measurements=None
  + : PMIOPort  Side=Left
  - : PMIOPort  Port=2  Side=Left
  Bat+ : PMIOPort  Port=3  Side=Right
  Bat- : PMIOPort  Port=4  Side=Right
  wires:
  Current Measurement1/1 -> Scope13/1, [I_Buck]
  PWM Generator (DC-DC)2/1 -> Scope1/1, [PWM_LIB1], NOT1/1
  NOT1/1 -> [PWM_LIB2]
  PID Controller1/1 -> PWM Generator (DC-DC)2/1
  Add1/1 -> PID Controller1/1
  [I_Buck] -> Add1/2
  PID Controller2/1 -> Add1/1
  [PWM_LIB1] -> IGBT/Diode1/1
  [PWM_LIB2] -> IGBT/Diode/1
  Constant2/1 -> Add2/2
  Vdc/1 -> Add2/1
  Add2/1 -> PID Controller2/1
  connections:
  Series RLC Branch2/LConn1 -- IGBT/Diode/LConn1 -- IGBT/Diode1/RConn1
  Current Measurement1/LConn1 -- Series RLC Branch2/RConn1
  Series RLC Branch4/RConn1 -- -/RConn1 -- IGBT/Diode/RConn1 -- Bat-/RConn1
  IGBT/Diode1/LConn1 -- +/RConn1
  Series RLC Branch4/LConn1 -- Current Measurement1/RConn1 -- Bat+/RConn1

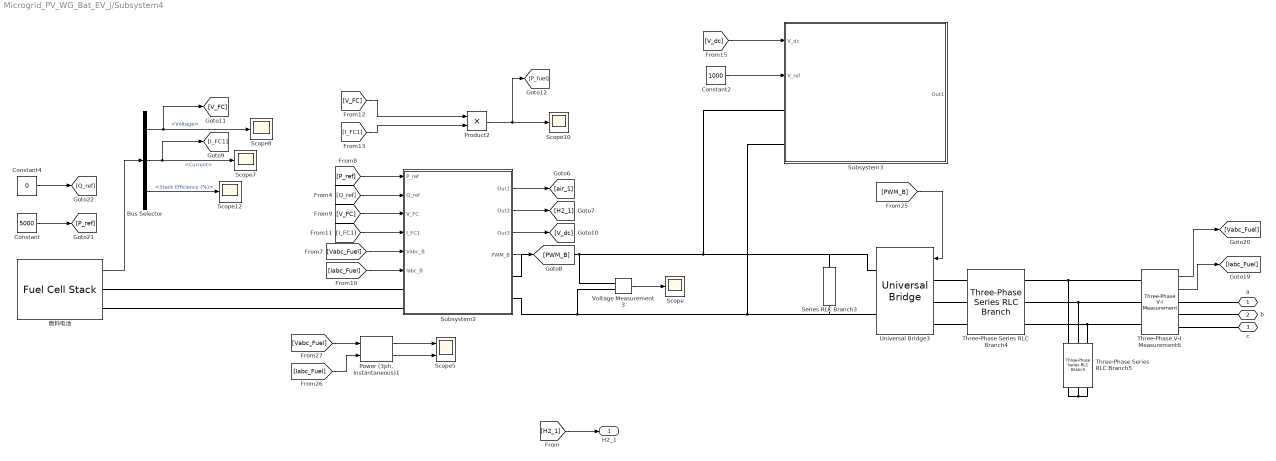
== system Microgrid_PV_WG_Bat_EV_j/Subsystem4 ==
  Bus Selector : BusSelector  OutputSignals=Voltage,Current,Stack Efficiency (%)
  Constant : Constant  Value=5000
  Constant2 : Constant  Value=1000
  Constant4 : Constant  Value=0
  "Power (3ph, Instantaneous)1" : spsPower3phInstantaneousLib/Power (3ph, Instantaneous)
  Product2 : Product
  Scope{,7..8,10,12} (5 alike) : Scope
  Scope5 : Scope  NumInputPorts=2
  Series RLC Branch3 : spsSeriesRLCBranchLib/Series RLC Branch  LConnTagsString=__new0  RConnTagsString=__new0  BranchType=RC  Resistance=0.05  Inductance=1e-3  SetiL0=off  InitialCurrent=0  Capacitance=7  Setx0=on  InitialVoltage=1000  Measurements=None
  Subsystem2 : Subsystem
  Subsystem3 : Subsystem
  Three-Phase Series RLC Branch4 : spsThreePhaseSeriesRLCBranchLib/Three-Phase Series RLC Branch  LConnTagsString=A|B|C  RConnTagsString=A|B|C  BranchType=L  Resistance=1  Inductance=3e-3  Capacitance=1e-6  Measurements=None
  Three-Phase Series RLC Branch5 : spsThreePhaseSeriesRLCBranchLib/Three-Phase Series RLC Branch  LConnTagsString=A|B|C  RConnTagsString=A|B|C  BranchType=RC  Resistance=0.01  Inductance=1e-3  Capacitance=3.2e-3  Measurements=None
  Three-Phase V-I Measurement6 : spsThreePhaseVIMeasurementLib/Three-Phase V-I Measurement  VoltageMeasurement=phase-to-ground  SetLabelV=off  LabelV=Vabc  Vpu=off  VpuLL=off  CurrentMeasurement=yes  SetLabelI=off  LabelI=Iabc  Ipu=off  Pbase=100e6  Vbase=500e3  OutputType=Complex  PhasorSimulation=off  PSBequivalent=0
  Universal Bridge3 : spsUniversalBridgeLib/Universal Bridge  Arms=3  SnubberResistance=1e5  SnubberCapacitance=inf  Device=IGBT / Diodes  Ron=1e-3  Lon=0  ForwardVoltages="[  0  0  ]"  ForwardVoltage=0  GTOparameters=[ 10e-6 , 20e-6 ]  IGBTparameters=[ 1e-6 , 2e-6 ]  Measurements=None  Measurements_2=None  converterType=Rectifier
  Voltage Measurement3 : spsVoltageMeasurementLib/Voltage Measurement  PhasorSimulation=off  OutputType=Complex  PSBequivalent=0
  燃料电池 : spsFuelCellStackLib/Fuel Cell Stack  PresetModel=PEMFC - 6 kW - 45 Vdc  FcType=0  Detailed=Detailed  Eoc=[65,63]  NomVI=[133.3,45]  EndVI=[225,37]  Nc=65  n=55  TOp=65  AirFr=300  SuppPress=[1.5,1]  Comp=[99.95,21,1]  SignX=off  SignY=off  FlowRateH2=on  FlowRateAir=on  SystemTemp=off  SystemPH2=off  SystemPAir=off  FCDyn=off  FC_tau=1  Peak_O2=80  V_Under=10
      settings: LibrarySourceBlock=sps_lib/Sources/Fuel Cell Stack
  a : PMIOPort  Side=Right
  b : PMIOPort  Port=2  Side=Right
  c : PMIOPort  Port=3  Side=Right
  H2_1 : Outport
  wires:
  "Power (3ph, Instantaneous)1"/1 -> Scope5/1
  [Q_ref] -> Subsystem2/2(Q_ref)
  [I_FC1] -> Subsystem2/4(I_FC1)
  Constant4/1 -> [Q_ref]
  Product2/1 -> [P_fuel], Scope10/1
  [I_FC1] -> Product2/2
  Subsystem2/1(Out1) -> [air_1]
  [V_FC] -> Product2/1
  [PWM_B] -> Universal Bridge3/1
  Bus Selector/1 -> [V_FC], Scope8/1  "<Voltage>"
  Three-Phase V-I Measurement6/1 -> [Vabc_Fuel]
  "Power (3ph, Instantaneous)1"/2 -> Scope5/2
  燃料电池/1 -> Bus Selector/1
  [Iabc_Fuel] -> "Power (3ph, Instantaneous)1"/2
  Subsystem2/3(Out3) -> [V_dc]
  Bus Selector/2 -> [I_FC1], Scope7/1  "<Current>"
  [P_ref] -> Subsystem2/1(P_ref)
  [Vabc_Fuel] -> Subsystem2/5(Vabc_B)
  [V_dc] -> Subsystem3/1(V_dc)
  Subsystem2/2(Out2) -> [H2_1]
  Constant/1 -> [P_ref]
  Bus Selector/3 -> Scope12/1  "<Stack Efficiency (%)>"
  [V_FC] -> Subsystem2/3(V_FC)
  Subsystem2/4(PWM_B) -> [PWM_B]
  [Vabc_Fuel] -> "Power (3ph, Instantaneous)1"/1
  [Iabc_Fuel] -> Subsystem2/6(Iabc_B)
  Voltage Measurement3/1 -> Scope/1
  Three-Phase V-I Measurement6/2 -> [Iabc_Fuel]
  Constant2/1 -> Subsystem3/2(V_ref)
  [H2_1] -> H2_1/1
  connections:
  Subsystem2/RConn2 -- Voltage Measurement3/LConn2 -- Universal Bridge3/RConn2 -- Series RLC Branch3/RConn1 -- Subsystem3/LConn2
  Subsystem2/LConn1 -- 燃料电池/RConn1
  Three-Phase Series RLC Branch5/LConn3 -- Three-Phase V-I Measurement6/LConn3 -- Three-Phase Series RLC Branch4/RConn3
  燃料电池/RConn2 -- Subsystem2/LConn2
  Three-Phase Series RLC Branch5/RConn3 -- Three-Phase Series RLC Branch5/RConn2 -- Three-Phase Series RLC Branch5/RConn1
  Voltage Measurement3/LConn1 -- Universal Bridge3/RConn1 -- Series RLC Branch3/LConn1 -- Subsystem3/LConn1 -- Subsystem2/RConn1
  Universal Bridge3/LConn3 -- Three-Phase Series RLC Branch4/LConn3
  Universal Bridge3/LConn2 -- Three-Phase Series RLC Branch4/LConn2
  Universal Bridge3/LConn1 -- Three-Phase Series RLC Branch4/LConn1
  Three-Phase Series RLC Branch5/LConn2 -- Three-Phase V-I Measurement6/LConn2 -- Three-Phase Series RLC Branch4/RConn2
  Three-Phase Series RLC Branch5/LConn1 -- Three-Phase V-I Measurement6/LConn1 -- Three-Phase Series RLC Branch4/RConn1
  Three-Phase V-I Measurement6/RConn3 -- c/RConn1
  Three-Phase V-I Measurement6/RConn2 -- b/RConn1
  Three-Phase V-I Measurement6/RConn1 -- a/RConn1

== system Microgrid_PV_WG_Bat_EV_j/WindTurbine ==
  note: 最佳叶尖速比下最大功率
  note: 风能利用系数
  note: 特定叶片最佳叶尖速比
  note: 电机实际转速
  note: 风速
  note: 直径
  note: 空气密度
  Wind speed : Inport
  Generator speed : Inport  Port=2
  Divide : Product  Inputs=/**
  Divide1 : Product  Inputs=/*
  Divide2 : Product  Inputs=*/
  Fcn : Fcn  Expr=1/(u(1)+0.08*u(2))-(0.035/(u(2)^3+1))
  Fcn1 : Fcn  Expr=0.5*u(1)*pi*u(2)^2*u(3)^3*u(4)
  Fcn2 : Fcn  Expr=0.5176*(116*u(2)-0.4*u(3)-5)*exp(-21*u(2))+0.006795*u(1)
  From : From
  Gain1 : Gain  Gain=0.5
  Gain2 : Gain  Gain=pi/30
  Gain3 : Gain  Gain=30/pi
  Goto : Goto
  Mux : Mux  Inputs=2
  Mux1 : Mux  Inputs=3
  Mux2 : Mux
  Product : Product
  Saturation : Saturate  UpperLimit=1e6  LowerLimit=1e-6
  Saturation1 : Saturate  UpperLimit=1e6  LowerLimit=1e-6
  Saturation2 : Saturate  UpperLimit=1e6  LowerLimit=1e-6
  Scope : Scope
  beta : Constant  Value=0
  density : Constant  Value=1.2
  diameter : Constant  Value=28
  lamda_nom : Constant  Value=8.1
  Tm : Outport
  n* : Outport  Port=2
  wires:
  Divide1/1 -> Mux1/1, Mux/1
  lamda_nom/1 -> Divide/3
  diameter/1 -> Gain1/1
  Generator speed/1 -> Gain2/1
  Gain2/1 -> Saturation/1
  Gain1/1 -> Mux2/2, Product/1, Divide/1
  Divide/1 -> Gain3/1
  beta/1 -> Mux1/3, Mux/2
  density/1 -> Mux2/1
  Mux/1 -> Fcn/1
  Mux2/1 -> Fcn1/1
  Gain3/1 -> n*/1
  Fcn/1 -> Mux1/2
  Product/1 -> Divide1/2
  Divide2/1 -> Tm/1
  Fcn1/1 -> Divide2/1  "Pm"
  Saturation1/1 -> Divide2/2
  Mux1/1 -> Fcn2/1
  Fcn2/1 -> Goto/1, Mux2/4  "Cp"
  Wind speed/1 -> Divide/2, Saturation2/1, Mux2/3
  Saturation/1 -> Saturation1/1, Product/2
  Saturation2/1 -> Divide1/1
  From/1 -> Scope/1
